simulink model "acm_robot_model_2017b"  (R2020a)
settings: Solver=ode4  StartTime=0.0  StopTime=30  FixedStep=1e-3  RelTol=1e-3
InitFcn:
  | acm_init
values from neighbouring files (symbols this model uses):
  alpha = 10*eye(2)    [acm_init.m]    (also in acm_init_final.m; calculating_YQ.m = 1)
  fd1 = 5.3    [acm_init.m]    (also in acm_init_final.m; calculating_YQ.m)
  fd2 = 1.1    [acm_init.m]    (also in acm_init_final.m; calculating_YQ.m)
  k = 1    [calculating_YQ.m]
  p1 = 3.473    [acm_init.m]    (also in acm_init_final.m; calculating_YQ.m)
  p2 = 0.196    [acm_init.m]    (also in acm_init_final.m; calculating_YQ.m)
  p3 = 0.242    [acm_init.m]    (also in acm_init_final.m; calculating_YQ.m)
settings Model: Creator=Tenghu  LastModifiedBy=User
settings SolverCC: ZeroCrossControl=EnableAll  AlgebraicLoopSolver=LineSearch
settings DataIOCC: SaveFormat=StructureWithTime
settings OptimizationCC: BlockReduction=off  BooleanDataType=off  LifeSpan=inf
settings DebuggingCC: SaveWithParameterizedLinksMsg=none  UnderspecifiedInitializationDetection=Classic  MergeDetectMultiDrivingBlocksExec=none  SignalResolutionControl=TryResolveAllWithWarning  AllowSymbolicDim=off  SFUnexpectedBacktrackingDiag=warning  SFNoUnconditionalDefaultTransitionDiag=warning  SFExecutionAtInitializationDiag=none  ArithmeticOperatorsInVariantConditions=warning
settings HardwareCC: ProdBitPerPointer=32  ProdBitPerSizeT=32  ProdBitPerPtrDiffT=32  ProdLargestAtomicFloat=None  ProdIntDivRoundTo=Undefined  ProdEndianess=Unspecified  ProdWordSize=32  ProdHWDeviceType=32-bit Generic  TargetBitPerPointer=64  TargetBitPerSizeT=64  TargetBitPerPtrDiffT=64  TargetLongLongMode=on  TargetIntDivRoundTo=Zero  TargetEndianess=LittleEndian  TargetWordSize=64  TargetHWDeviceType=MATLAB Host  ProdEqTarget=off
settings ModelReferenceCC: PropagateSignalLabelsOutOfModel=off
settings SFSimCC: SimUseLocalCustomCode=off  CustomCodeUndefinedFunction=UseInterfaceOnly
settings RTWCC: RTWUseLocalCustomCode=off
settings CodeAppCC: StateflowObjectComments=on
settings GRTTargetCC: TargetLangStandard=C89/C90 (ANSI)
settings ConfigComp: CovMetricSettings=dw  CovHtmlReporting=on  CovSaveCumulativeToWorkspaceVar=on  CovSaveSingleToWorkspaceVar=on  CovExternalEMLEnable=off  CovSFcnEnable=off

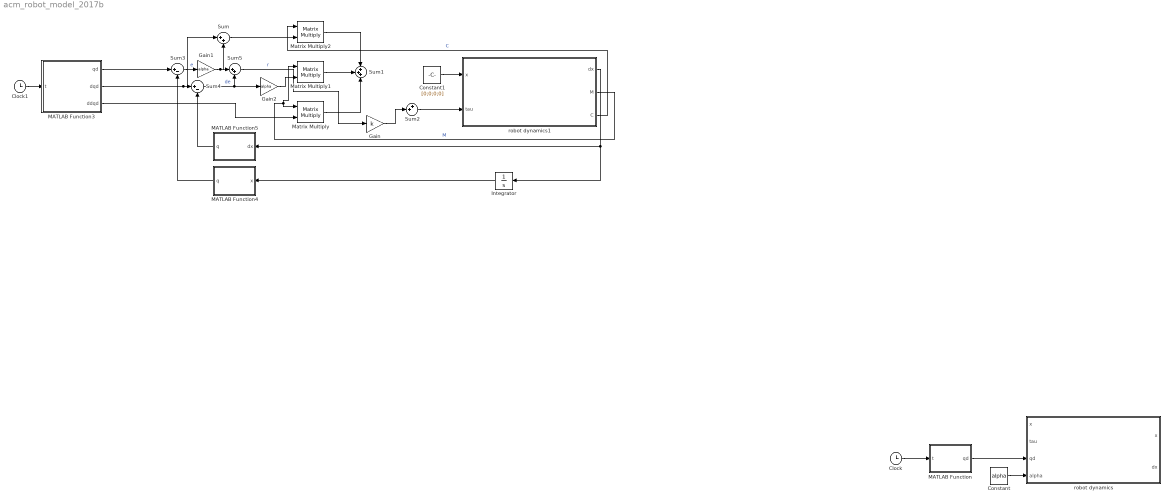
== system acm_robot_model_2017b ==
  Clock : Clock
  Clock1 : Clock
  Constant : Constant  Value=alpha
  Constant1 : Constant  Value=[0;0;0;0]
  Gain : Gain  Gain=k
  Gain1 : Gain  Gain=alpha
  Gain2 : Gain  Gain=alpha
  Integrator : Integrator
  MATLAB Function : MATLAB Function  TreatAsAtomicUnit=on
  MATLAB Function3 : MATLAB Function  TreatAsAtomicUnit=on
  MATLAB Function4 : MATLAB Function  TreatAsAtomicUnit=on
  MATLAB Function5 : MATLAB Function  TreatAsAtomicUnit=on
  Matrix Multiply : Product  Multiplication=Matrix(*)
  Matrix Multiply1 : Product  Multiplication=Matrix(*)
  Matrix Multiply2 : Product  Multiplication=Matrix(*)
  Sum : Sum  Inputs=|++
  Sum1 : Sum  Inputs=+++
  Sum2 : Sum  Inputs=++|
  Sum3 : Sum  Inputs=|+-
  Sum4 : Sum  Inputs=|+-
  Sum5 : Sum  Inputs=|++
  robot dynamics : MATLAB Function  TreatAsAtomicUnit=on
  robot dynamics1 : MATLAB Function  TreatAsAtomicUnit=on
  wires:
  Clock/1 -> MATLAB Function/1(t)
  MATLAB Function4/1(q) -> Sum3/2
  Sum3/1 -> Gain1/1  "e"
  Gain1/1 -> Sum/2, Sum5/1
  MATLAB Function5/1(q) -> Sum4/2
  Sum4/1 -> Gain2/1, Sum5/2  "de"
  MATLAB Function3/1(qd) -> Sum3/1
  MATLAB Function3/2(dqd) -> Sum/1, Sum4/1
  Clock1/1 -> MATLAB Function3/1(t)
  MATLAB Function/1(qd) -> robot dynamics/3(qd)
  Constant/1 -> robot dynamics/4(alpha)
  Sum5/1 -> Gain/1  "r"
  Integrator/1 -> MATLAB Function4/1(x)
  robot dynamics1/1(dx) -> Integrator/1, MATLAB Function5/1(dx)
  robot dynamics1/2(M) -> Matrix Multiply1/1, Matrix Multiply/1  "M"
  MATLAB Function3/3(ddqd) -> Matrix Multiply/2
  Gain2/1 -> Matrix Multiply1/2
  robot dynamics1/3(C) -> Matrix Multiply2/1  "C"
  Sum/1 -> Matrix Multiply2/2
  Matrix Multiply1/1 -> Sum1/2
  Matrix Multiply2/1 -> Sum1/1
  Matrix Multiply/1 -> Sum1/3
  Gain/1 -> Sum2/2
  Sum2/1 -> robot dynamics1/2(tau)
  Constant1/1 -> robot dynamics1/1(x)

== matlab function acm_robot_model_2017b/MATLAB Function ==
  data: t input; qd output
function qd = desired_traj(t)
qd=zeros(2,1);
qd(1)=sin(3*t);
qd(2)=2*cos(t);
end

== matlab function acm_robot_model_2017b/robot dynamics ==
  data: x output; x input; dx output; tau input; p1 parameter; p2 parameter; p3 parameter; fd1 parameter; fd2 parameter; qd input; alpha input
% *************************************************************************
%                        2-Link Manipulator Dynamics                      *
% *************************************************************************

function [x,dx] = fcn_twoLinkDynamics(x, tau, p1, p2, p3, fd1, fd2, qd, alpha)
    q1  = x(1);
    dq1 = x(2);
    q2  = x(3);
    dq2 = x(4);
    
    M      = zeros(2,2);
    M(1,1) = p1 + 2*p3*cos(q2);
    M(1,2) = p2 + p3*cos(q2);
    M(2,1) = p2 + p3*cos(q2);
    M(2,2) = p2;

    C      = zeros(2,2);
    C(1,1) = -p3*sin(q2)*dq2;
    C(1,2) = -p3*sin(q2)*(dq1+dq2);
    C(2,1) = p3*sin(q2)*dq1;
    C(2,2) = 0;

    Fd     = diag([fd1 fd2]);

    % The system without bounded disturbances =============================
    ddq = M\(tau - C*[dq1;dq2] - Fd*[dq1;dq2]);
    dx  = [dq1; ddq(1); dq2; ddq(2)];
    e   = qd-[q1;q2];
    de  = jacobian(e,t);
    dde = jacobian(de,t);
    r   = e-alpha*de;
    dr  = de-alpha*dde;
    
end

== matlab function acm_robot_model_2017b/MATLAB Function3 ==
  data: t input; qd output; dqd output; ddqd output
function [qd,dqd,ddqd] = desired_traj(t)
qd=zeros(2,1);
qd(1)=sin(3*t);
qd(2)=2*cos(t);
dqd=zeros(2,1);
dqd(1)=3*cos(3*t);
dqd(2)=-2*sin(t);
ddqd=zeros(2,1);
ddqd(1)=-9*sin(3*t);
ddqd(2)=-2*cos(t);
end

== matlab function acm_robot_model_2017b/MATLAB Function4 ==
  data: x input; q output
function q=takeq(x)
q=zeros(2,1);
q(1)=x(1);
q(2)=x(3);
end

== matlab function acm_robot_model_2017b/MATLAB Function5 ==
  data: dx input; q output
function q=takedq(dx)
q=zeros(2,1);
q(1)=x(1);
q(2)=x(3);
end

== matlab function acm_robot_model_2017b/robot dynamics1 ==
  data: x input; dx output; tau input; p1 parameter; p2 parameter; p3 parameter; fd1 parameter; fd2 parameter; M output; C output
% *************************************************************************
%                        2-Link Manipulator Dynamics                      *
% *************************************************************************

function [dx,M,C] = fcn_twoLinkDynamics(x, tau, p1, p2, p3, fd1, fd2)
    q1  = x(1);
    dq1 = x(2);
    q2  = x(3);
    dq2 = x(4);
    
    M      = zeros(2,2);
    M(1,1) = p1 + 2*p3*cos(q2);
    M(1,2) = p2 + p3*cos(q2);
    M(2,1) = p2 + p3*cos(q2);
    M(2,2) = p2;

    C      = zeros(2,2);
    C(1,1) = -p3*sin(q2)*dq2;
    C(1,2) = -p3*sin(q2)*(dq1+dq2);
    C(2,1) = p3*sin(q2)*dq1;
    C(2,2) = 0;

    Fd     = diag([fd1 fd2]);

    % The system without bounded disturbances =============================
    ddq = M\(tau - C*[dq1;dq2] - Fd*[dq1;dq2]);
    dx  = [dq1; ddq(1); dq2; ddq(2)];
end
